simulink model "TST_Tra_RtnIntfc"  (R2016b)
settings: Solver=FixedStepDiscrete  StartTime=0.0  StopTime=simTime  FixedStep=sampleTime  RelTol=1e-3
values from neighbouring files (symbols this model uses):
  testCase = 1    [initTST_Tra_RtnIntfc_001.m]    (also in initTST_Tra_RtnIntfc_002.m = 2)
libraries: simulink x9, UnitTest_Lib x6
settings Model: Creator=zhengjinyan  LastModifiedBy=zhengjinyan
settings DebuggingCC: SignalRangeChecking=error

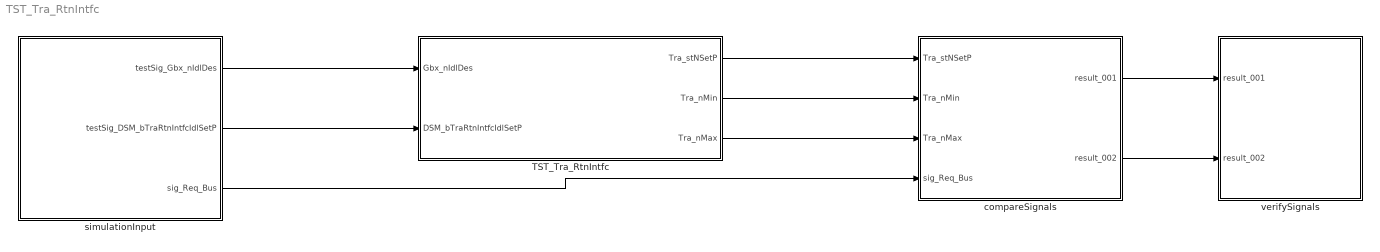
== system TST_Tra_RtnIntfc ==
  TST_Tra_RtnIntfc : Subsystem
  compareSignals : Subsystem
  simulationInput : Subsystem
  verifySignals : Subsystem
  wires:
  simulationInput/1(testSig_Gbx_nIdlDes) -> TST_Tra_RtnIntfc/1(Gbx_nIdlDes)
  simulationInput/2(testSig_DSM_bTraRtnIntfcIdlSetP) -> TST_Tra_RtnIntfc/2(DSM_bTraRtnIntfcIdlSetP)
  TST_Tra_RtnIntfc/1(Tra_stNSetP) -> compareSignals/1(Tra_stNSetP)
  TST_Tra_RtnIntfc/2(Tra_nMin) -> compareSignals/2(Tra_nMin)
  TST_Tra_RtnIntfc/3(Tra_nMax) -> compareSignals/3(Tra_nMax)
  simulationInput/3(sig_Req_Bus) -> compareSignals/4(sig_Req_Bus)
  compareSignals/1(result_001) -> verifySignals/1(result_001)
  compareSignals/2(result_002) -> verifySignals/2(result_002)

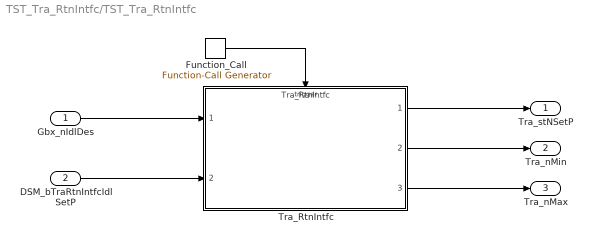
== system TST_Tra_RtnIntfc/TST_Tra_RtnIntfc ==
  Gbx_nIdlDes : Inport
  DSM_bTraRtnIntfcIdlSetP : Inport  Port=2
  Function_Call : simulink/Ports & Subsystems/Function-Call Generator  sample_time=sampleTime  numberOfIterations=1
  Tra_RtnIntfc : ModelReference  ModelNameDialog=Tra_RtnIntfc  SimulationMode=Normal  ModelReferenceVersion=1.13  TriggerPortName=function  TriggerPortTriggerType=function-call  TriggerPortStatesWhenEnabling=held
  Tra_stNSetP : Outport
  Tra_nMin : Outport  Port=2
  Tra_nMax : Outport  Port=3
  wires:
  Function_Call/1 -> Tra_RtnIntfc/Trigger
  Gbx_nIdlDes/1 -> Tra_RtnIntfc/1
  DSM_bTraRtnIntfcIdlSetP/1 -> Tra_RtnIntfc/2
  Tra_RtnIntfc/1 -> Tra_stNSetP/1
  Tra_RtnIntfc/2 -> Tra_nMin/1
  Tra_RtnIntfc/3 -> Tra_nMax/1

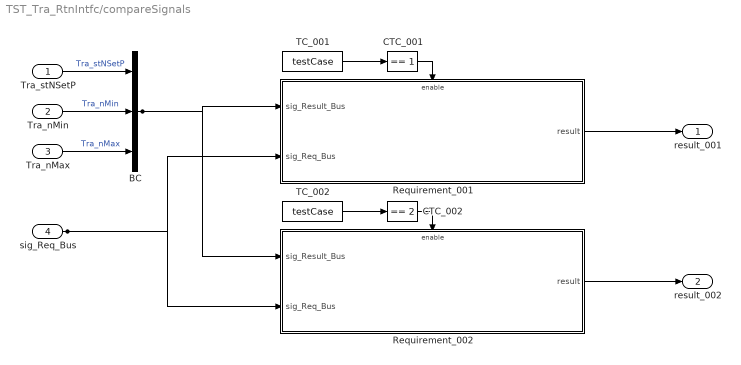
== system TST_Tra_RtnIntfc/compareSignals ==
  Tra_stNSetP : Inport
  Tra_nMin : Inport  Port=2
  Tra_nMax : Inport  Port=3
  sig_Req_Bus : Inport  Port=4
  BC : BusCreator  Inputs=3
  CTC_001 : simulink/Logic and Bit Operations/Compare To Constant  relop===  const=1  OutDataTypeStr=boolean
  CTC_002 : simulink/Logic and Bit Operations/Compare To Constant  relop===  const=2  OutDataTypeStr=boolean
  Requirement_001 : Subsystem
  Requirement_002 : Subsystem
  TC_001 : Constant  Value=testCase
  TC_002 : Constant  Value=testCase
  result_001 : Outport
  result_002 : Outport  Port=2
  wires:
  Tra_stNSetP/1 -> BC/1  "Tra_stNSetP"
  Tra_nMin/1 -> BC/2  "Tra_nMin"
  Tra_nMax/1 -> BC/3  "Tra_nMax"
  TC_001/1 -> CTC_001/1
  CTC_001/1 -> Requirement_001/Enable
  sig_Req_Bus/1 -> Requirement_001/2(sig_Req_Bus), Requirement_002/2(sig_Req_Bus)
  BC/1 -> Requirement_001/1(sig_Result_Bus), Requirement_002/1(sig_Result_Bus)
  Requirement_001/1(result) -> result_001/1
  TC_002/1 -> CTC_002/1
  CTC_002/1 -> Requirement_002/Enable
  Requirement_002/1(result) -> result_002/1

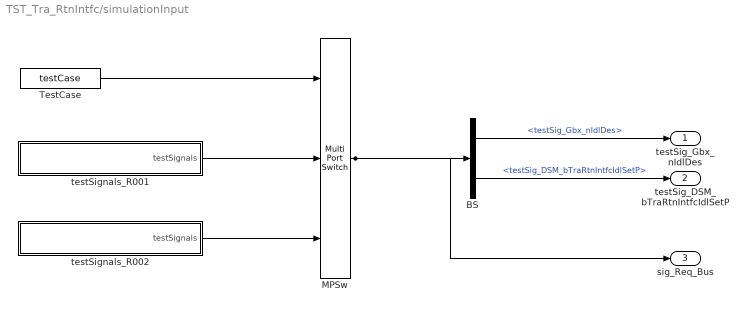
== system TST_Tra_RtnIntfc/simulationInput ==
  BS : BusSelector  OutputSignals=testSig_Gbx_nIdlDes,testSig_DSM_bTraRtnIntfcIdlSetP
  MPSw : MultiPortSwitch  Inputs=2  SaturateOnIntegerOverflow=on  InputSameDT=on
  TestCase : Constant  Value=testCase
  testSignals_R001 : Subsystem
  testSignals_R002 : Subsystem
  testSig_Gbx_nIdlDes : Outport
  testSig_DSM_bTraRtnIntfcIdlSetP : Outport  Port=2
  sig_Req_Bus : Outport  Port=3
  wires:
  BS/1 -> testSig_Gbx_nIdlDes/1  "<testSig_Gbx_nIdlDes>"
  BS/2 -> testSig_DSM_bTraRtnIntfcIdlSetP/1  "<testSig_DSM_bTraRtnIntfcIdlSetP>"
  MPSw/1 -> BS/1, sig_Req_Bus/1
  TestCase/1 -> MPSw/1
  testSignals_R001/1(testSignals) -> MPSw/2
  testSignals_R002/1(testSignals) -> MPSw/3

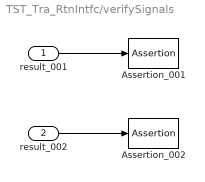
== system TST_Tra_RtnIntfc/verifySignals ==
  result_001 : Inport
  result_002 : Inport  Port=2
  Assertion_001 : Assertion  Enabled=off
  Assertion_002 : Assertion  Enabled=off
  wires:
  result_001/1 -> Assertion_001/1
  result_002/1 -> Assertion_002/1

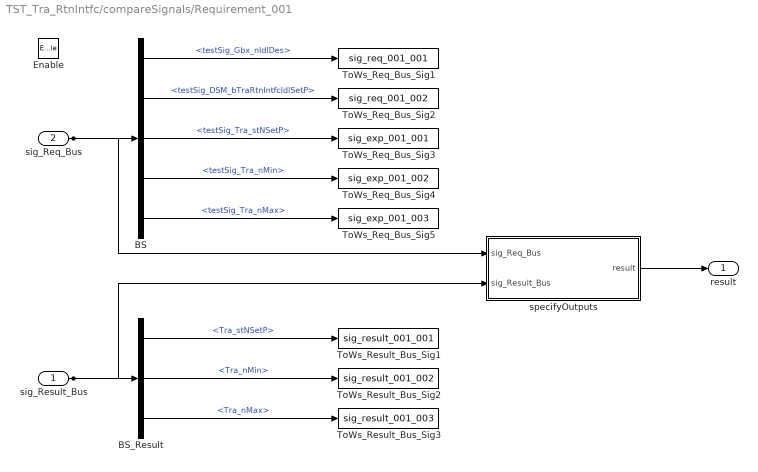
== system TST_Tra_RtnIntfc/compareSignals/Requirement_001 ==
  sig_Result_Bus : Inport
  sig_Req_Bus : Inport  Port=2
  Enable : EnablePort
  BS : BusSelector  OutputSignals=testSig_Gbx_nIdlDes,testSig_DSM_bTraRtnIntfcIdlSetP,testSig_Tra_stNSetP,testSig_Tra_nMin,testSig_Tra_nMax
  BS_Result : BusSelector  OutputSignals=Tra_stNSetP,Tra_nMin,Tra_nMax
  ToWs_Req_Bus_Sig1 : ToWorkspace  VariableName=sig_req_001_001  SaveFormat=Structure With Time
  ToWs_Req_Bus_Sig2 : ToWorkspace  VariableName=sig_req_001_002  SaveFormat=Structure With Time
  ToWs_Req_Bus_Sig3 : ToWorkspace  VariableName=sig_exp_001_001  SaveFormat=Structure With Time
  ToWs_Req_Bus_Sig4 : ToWorkspace  VariableName=sig_exp_001_002  SaveFormat=Structure With Time
  ToWs_Req_Bus_Sig5 : ToWorkspace  VariableName=sig_exp_001_003  SaveFormat=Structure With Time
  ToWs_Result_Bus_Sig1 : ToWorkspace  VariableName=sig_result_001_001  SaveFormat=Structure With Time
  ToWs_Result_Bus_Sig2 : ToWorkspace  VariableName=sig_result_001_002  SaveFormat=Structure With Time
  ToWs_Result_Bus_Sig3 : ToWorkspace  VariableName=sig_result_001_003  SaveFormat=Structure With Time
  specifyOutputs : Subsystem
  result : Outport
  wires:
  sig_Req_Bus/1 -> BS/1, specifyOutputs/1(sig_Req_Bus)
  BS/1 -> ToWs_Req_Bus_Sig1/1  "<testSig_Gbx_nIdlDes>"
  BS/2 -> ToWs_Req_Bus_Sig2/1  "<testSig_DSM_bTraRtnIntfcIdlSetP>"
  BS/3 -> ToWs_Req_Bus_Sig3/1  "<testSig_Tra_stNSetP>"
  BS/4 -> ToWs_Req_Bus_Sig4/1  "<testSig_Tra_nMin>"
  BS/5 -> ToWs_Req_Bus_Sig5/1  "<testSig_Tra_nMax>"
  sig_Result_Bus/1 -> BS_Result/1, specifyOutputs/2(sig_Result_Bus)
  BS_Result/1 -> ToWs_Result_Bus_Sig1/1  "<Tra_stNSetP>"
  BS_Result/2 -> ToWs_Result_Bus_Sig2/1  "<Tra_nMin>"
  BS_Result/3 -> ToWs_Result_Bus_Sig3/1  "<Tra_nMax>"
  specifyOutputs/1(result) -> result/1

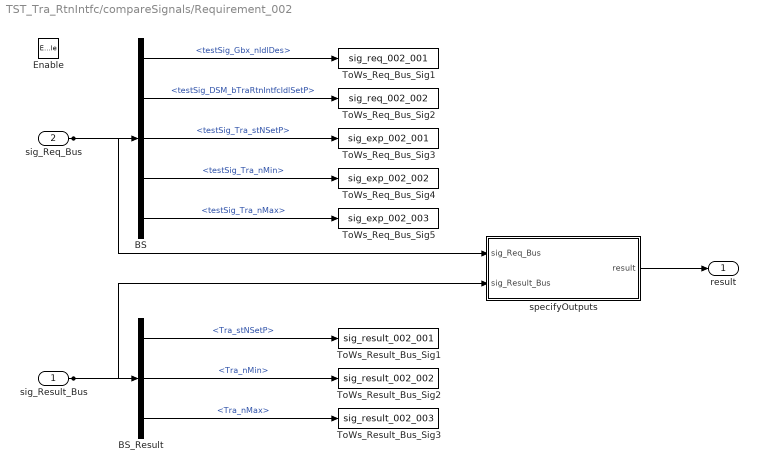
== system TST_Tra_RtnIntfc/compareSignals/Requirement_002 ==
  sig_Result_Bus : Inport
  sig_Req_Bus : Inport  Port=2
  Enable : EnablePort
  BS : BusSelector  OutputSignals=testSig_Gbx_nIdlDes,testSig_DSM_bTraRtnIntfcIdlSetP,testSig_Tra_stNSetP,testSig_Tra_nMin,testSig_Tra_nMax
  BS_Result : BusSelector  OutputSignals=Tra_stNSetP,Tra_nMin,Tra_nMax
  ToWs_Req_Bus_Sig1 : ToWorkspace  VariableName=sig_req_002_001  SaveFormat=Structure With Time
  ToWs_Req_Bus_Sig2 : ToWorkspace  VariableName=sig_req_002_002  SaveFormat=Structure With Time
  ToWs_Req_Bus_Sig3 : ToWorkspace  VariableName=sig_exp_002_001  SaveFormat=Structure With Time
  ToWs_Req_Bus_Sig4 : ToWorkspace  VariableName=sig_exp_002_002  SaveFormat=Structure With Time
  ToWs_Req_Bus_Sig5 : ToWorkspace  VariableName=sig_exp_002_003  SaveFormat=Structure With Time
  ToWs_Result_Bus_Sig1 : ToWorkspace  VariableName=sig_result_002_001  SaveFormat=Structure With Time
  ToWs_Result_Bus_Sig2 : ToWorkspace  VariableName=sig_result_002_002  SaveFormat=Structure With Time
  ToWs_Result_Bus_Sig3 : ToWorkspace  VariableName=sig_result_002_003  SaveFormat=Structure With Time
  specifyOutputs : Subsystem
  result : Outport
  wires:
  sig_Req_Bus/1 -> BS/1, specifyOutputs/1(sig_Req_Bus)
  BS/1 -> ToWs_Req_Bus_Sig1/1  "<testSig_Gbx_nIdlDes>"
  BS/2 -> ToWs_Req_Bus_Sig2/1  "<testSig_DSM_bTraRtnIntfcIdlSetP>"
  BS/3 -> ToWs_Req_Bus_Sig3/1  "<testSig_Tra_stNSetP>"
  BS/4 -> ToWs_Req_Bus_Sig4/1  "<testSig_Tra_nMin>"
  BS/5 -> ToWs_Req_Bus_Sig5/1  "<testSig_Tra_nMax>"
  sig_Result_Bus/1 -> BS_Result/1, specifyOutputs/2(sig_Result_Bus)
  BS_Result/1 -> ToWs_Result_Bus_Sig1/1  "<Tra_stNSetP>"
  BS_Result/2 -> ToWs_Result_Bus_Sig2/1  "<Tra_nMin>"
  BS_Result/3 -> ToWs_Result_Bus_Sig3/1  "<Tra_nMax>"
  specifyOutputs/1(result) -> result/1

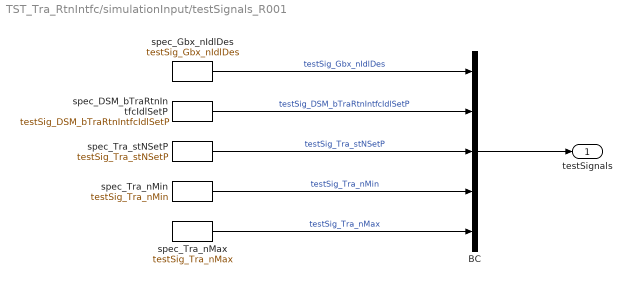
== system TST_Tra_RtnIntfc/simulationInput/testSignals_R001 ==
  BC : BusCreator  Inputs=5
  spec_DSM_bTraRtnIntfcIdlSetP : FromWorkspace  VariableName=testSig_DSM_bTraRtnIntfcIdlSetP  Interpolate=off  OutputAfterFinalValue=Holding final value
  spec_Gbx_nIdlDes : FromWorkspace  VariableName=testSig_Gbx_nIdlDes  Interpolate=off  OutputAfterFinalValue=Holding final value
  spec_Tra_nMax : FromWorkspace  VariableName=testSig_Tra_nMax  Interpolate=off  OutputAfterFinalValue=Holding final value
  spec_Tra_nMin : FromWorkspace  VariableName=testSig_Tra_nMin  Interpolate=off  OutputAfterFinalValue=Holding final value
  spec_Tra_stNSetP : FromWorkspace  VariableName=testSig_Tra_stNSetP  Interpolate=off  OutputAfterFinalValue=Holding final value
  testSignals : Outport
  wires:
  BC/1 -> testSignals/1
  spec_Gbx_nIdlDes/1 -> BC/1  "testSig_Gbx_nIdlDes"
  spec_DSM_bTraRtnIntfcIdlSetP/1 -> BC/2  "testSig_DSM_bTraRtnIntfcIdlSetP"
  spec_Tra_stNSetP/1 -> BC/3  "testSig_Tra_stNSetP"
  spec_Tra_nMin/1 -> BC/4  "testSig_Tra_nMin"
  spec_Tra_nMax/1 -> BC/5  "testSig_Tra_nMax"

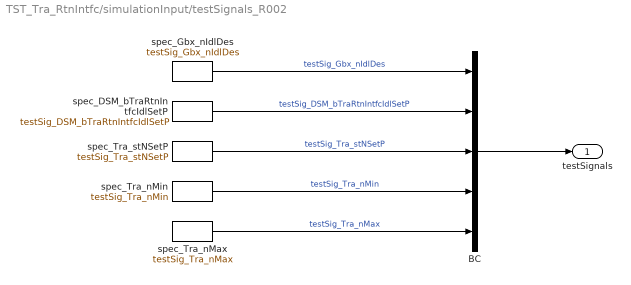
== system TST_Tra_RtnIntfc/simulationInput/testSignals_R002 ==
  BC : BusCreator  Inputs=5
  spec_DSM_bTraRtnIntfcIdlSetP : FromWorkspace  VariableName=testSig_DSM_bTraRtnIntfcIdlSetP  Interpolate=off  OutputAfterFinalValue=Holding final value
  spec_Gbx_nIdlDes : FromWorkspace  VariableName=testSig_Gbx_nIdlDes  Interpolate=off  OutputAfterFinalValue=Holding final value
  spec_Tra_nMax : FromWorkspace  VariableName=testSig_Tra_nMax  Interpolate=off  OutputAfterFinalValue=Holding final value
  spec_Tra_nMin : FromWorkspace  VariableName=testSig_Tra_nMin  Interpolate=off  OutputAfterFinalValue=Holding final value
  spec_Tra_stNSetP : FromWorkspace  VariableName=testSig_Tra_stNSetP  Interpolate=off  OutputAfterFinalValue=Holding final value
  testSignals : Outport
  wires:
  BC/1 -> testSignals/1
  spec_Gbx_nIdlDes/1 -> BC/1  "testSig_Gbx_nIdlDes"
  spec_DSM_bTraRtnIntfcIdlSetP/1 -> BC/2  "testSig_DSM_bTraRtnIntfcIdlSetP"
  spec_Tra_stNSetP/1 -> BC/3  "testSig_Tra_stNSetP"
  spec_Tra_nMin/1 -> BC/4  "testSig_Tra_nMin"
  spec_Tra_nMax/1 -> BC/5  "testSig_Tra_nMax"

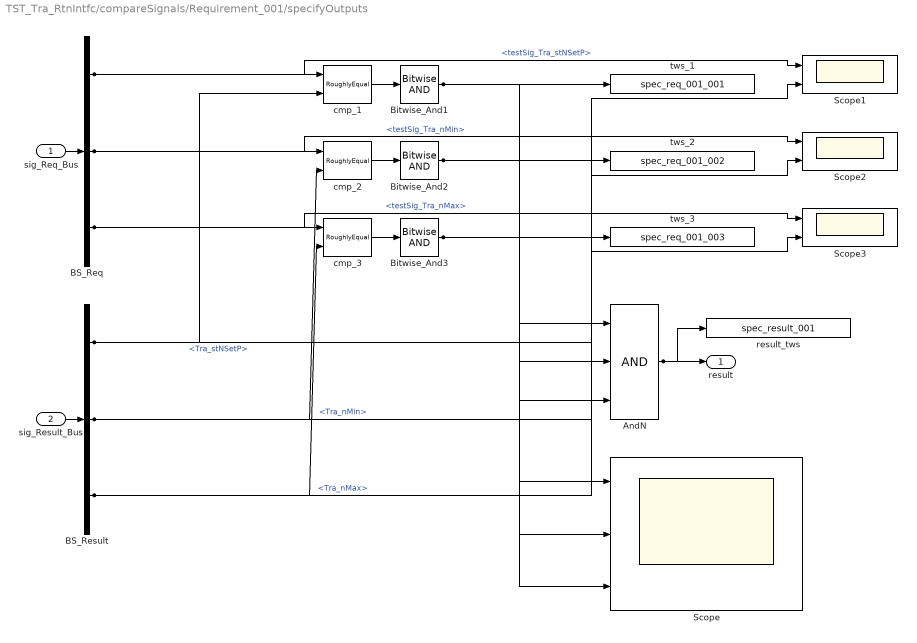
== system TST_Tra_RtnIntfc/compareSignals/Requirement_001/specifyOutputs ==
  sig_Req_Bus : Inport
  sig_Result_Bus : Inport  Port=2
  AndN : Logic  Inputs=3
  BS_Req : BusSelector  OutputSignals=testSig_Tra_stNSetP,testSig_Tra_nMin,testSig_Tra_nMax
  BS_Result : BusSelector  OutputSignals=Tra_stNSetP,Tra_nMin,Tra_nMax
  Bitwise_And1 : simulink/Logic and Bit Operations/Bitwise Operator  logicop=AND  UseBitMask=off  BitMask=bin2dec('11011001')  BitMaskRealWorld=Stored Integer
  Bitwise_And2 : simulink/Logic and Bit Operations/Bitwise Operator  logicop=AND  UseBitMask=off  BitMask=bin2dec('11011001')  BitMaskRealWorld=Stored Integer
  Bitwise_And3 : simulink/Logic and Bit Operations/Bitwise Operator  logicop=AND  UseBitMask=off  BitMask=bin2dec('11011001')  BitMaskRealWorld=Stored Integer
  Scope : Scope  NumInputPorts=3
  Scope1 : Scope  NumInputPorts=2
  Scope2 : Scope  NumInputPorts=2
  Scope3 : Scope  NumInputPorts=2
  cmp_1 : UnitTest_Lib/RoughlyEqual  slope=0.1
  cmp_2 : UnitTest_Lib/RoughlyEqual  slope=0.1
  cmp_3 : UnitTest_Lib/RoughlyEqual  slope=0.1
  result_tws : ToWorkspace  VariableName=spec_result_001
  tws_1 : ToWorkspace  VariableName=spec_req_001_001
  tws_2 : ToWorkspace  VariableName=spec_req_001_002
  tws_3 : ToWorkspace  VariableName=spec_req_001_003
  result : Outport
  wires:
  sig_Req_Bus/1 -> BS_Req/1
  sig_Result_Bus/1 -> BS_Result/1
  AndN/1 -> result/1, result_tws/1
  BS_Req/1 -> cmp_1/1, Scope1/1  "<testSig_Tra_stNSetP>"
  BS_Result/1 -> cmp_1/2, Scope1/2  "<Tra_stNSetP>"
  cmp_1/1 -> Bitwise_And1/1
  Bitwise_And1/1 -> tws_1/1, AndN/1, Scope/1
  BS_Req/2 -> cmp_2/1, Scope2/1  "<testSig_Tra_nMin>"
  BS_Result/2 -> cmp_2/2, Scope2/2  "<Tra_nMin>"
  cmp_2/1 -> Bitwise_And2/1
  Bitwise_And2/1 -> tws_2/1, AndN/2, Scope/2
  BS_Req/3 -> cmp_3/1, Scope3/1  "<testSig_Tra_nMax>"
  BS_Result/3 -> cmp_3/2, Scope3/2  "<Tra_nMax>"
  cmp_3/1 -> Bitwise_And3/1
  Bitwise_And3/1 -> tws_3/1, AndN/3, Scope/3

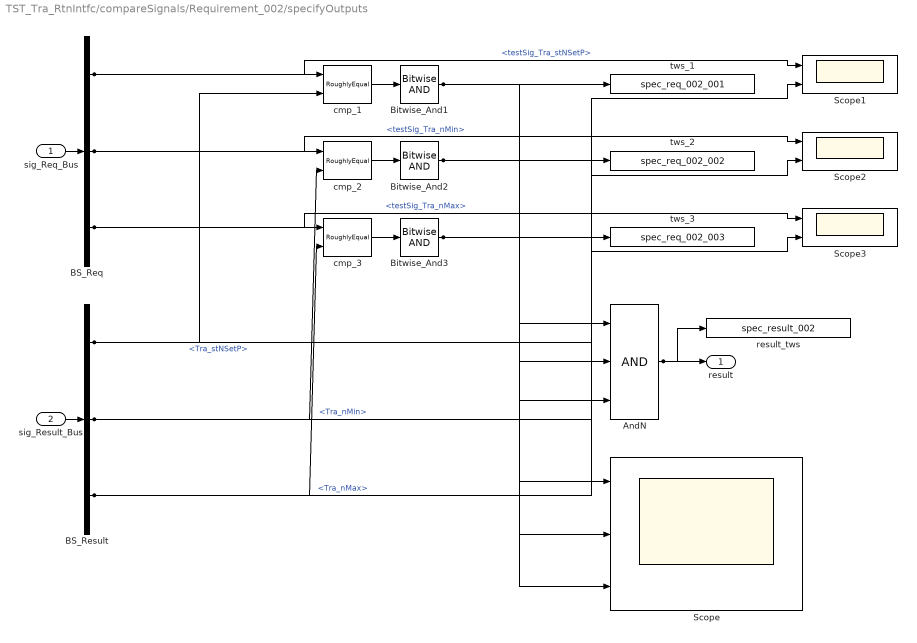
== system TST_Tra_RtnIntfc/compareSignals/Requirement_002/specifyOutputs ==
  sig_Req_Bus : Inport
  sig_Result_Bus : Inport  Port=2
  AndN : Logic  Inputs=3
  BS_Req : BusSelector  OutputSignals=testSig_Tra_stNSetP,testSig_Tra_nMin,testSig_Tra_nMax
  BS_Result : BusSelector  OutputSignals=Tra_stNSetP,Tra_nMin,Tra_nMax
  Bitwise_And1 : simulink/Logic and Bit Operations/Bitwise Operator  logicop=AND  UseBitMask=off  BitMask=bin2dec('11011001')  BitMaskRealWorld=Stored Integer
  Bitwise_And2 : simulink/Logic and Bit Operations/Bitwise Operator  logicop=AND  UseBitMask=off  BitMask=bin2dec('11011001')  BitMaskRealWorld=Stored Integer
  Bitwise_And3 : simulink/Logic and Bit Operations/Bitwise Operator  logicop=AND  UseBitMask=off  BitMask=bin2dec('11011001')  BitMaskRealWorld=Stored Integer
  Scope : Scope  NumInputPorts=3
  Scope1 : Scope  NumInputPorts=2
  Scope2 : Scope  NumInputPorts=2
  Scope3 : Scope  NumInputPorts=2
  cmp_1 : UnitTest_Lib/RoughlyEqual  slope=0.1
  cmp_2 : UnitTest_Lib/RoughlyEqual  slope=0.1
  cmp_3 : UnitTest_Lib/RoughlyEqual  slope=0.1
  result_tws : ToWorkspace  VariableName=spec_result_002
  tws_1 : ToWorkspace  VariableName=spec_req_002_001
  tws_2 : ToWorkspace  VariableName=spec_req_002_002
  tws_3 : ToWorkspace  VariableName=spec_req_002_003
  result : Outport
  wires:
  sig_Req_Bus/1 -> BS_Req/1
  sig_Result_Bus/1 -> BS_Result/1
  AndN/1 -> result/1, result_tws/1
  BS_Req/1 -> cmp_1/1, Scope1/1  "<testSig_Tra_stNSetP>"
  BS_Result/1 -> cmp_1/2, Scope1/2  "<Tra_stNSetP>"
  cmp_1/1 -> Bitwise_And1/1
  Bitwise_And1/1 -> tws_1/1, AndN/1, Scope/1
  BS_Req/2 -> cmp_2/1, Scope2/1  "<testSig_Tra_nMin>"
  BS_Result/2 -> cmp_2/2, Scope2/2  "<Tra_nMin>"
  cmp_2/1 -> Bitwise_And2/1
  Bitwise_And2/1 -> tws_2/1, AndN/2, Scope/2
  BS_Req/3 -> cmp_3/1, Scope3/1  "<testSig_Tra_nMax>"
  BS_Result/3 -> cmp_3/2, Scope3/2  "<Tra_nMax>"
  cmp_3/1 -> Bitwise_And3/1
  Bitwise_And3/1 -> tws_3/1, AndN/3, Scope/3
